simulink library "THV2THB"  (Simulink 8.2)
settings: Solver=ode45  StartTime=0.0  StopTime=10.0  RelTol=1e-3
settings Model: Creator=lena.frank  LastModifiedBy=drhf

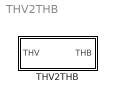
== system THV2THB ==
  THV2THB : Subsystem  InitFcn=load('THB.mat');  mask(THV2THB){}
      mask help: This block converts the old Thermo-Hydraulic-Vector to the Thermo-Hydraulic-Bus.
      mask Help: web(fullfile(path_carnot('help'),'THV2THB.html'),'-helpbrowser')

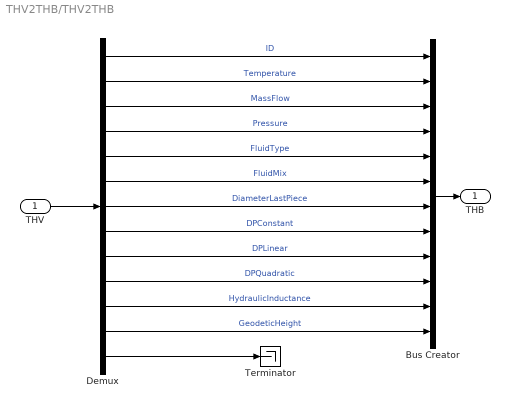
== system THV2THB/THV2THB ==
  THV : Inport
  Bus Creator : BusCreator  Inputs=12  OutDataTypeStr=Bus: THB
  Demux : Demux  Outputs=[1 1 1 1 1 1 1 1 1 1 1 1 8]
  Terminator : Terminator
  THB : Outport
  wires:
  Demux/11 -> Bus Creator/11  "HydraulicInductance"
  THV/1 -> Demux/1
  Demux/2 -> Bus Creator/2  "Temperature"
  Demux/1 -> Bus Creator/1  "ID"
  Demux/3 -> Bus Creator/3  "MassFlow"
  Demux/4 -> Bus Creator/4  "Pressure"
  Bus Creator/1 -> THB/1
  Demux/5 -> Bus Creator/5  "FluidType"
  Demux/6 -> Bus Creator/6  "FluidMix"
  Demux/7 -> Bus Creator/7  "DiameterLastPiece"
  Demux/8 -> Bus Creator/8  "DPConstant"
  Demux/9 -> Bus Creator/9  "DPLinear"
  Demux/10 -> Bus Creator/10  "DPQuadratic"
  Demux/12 -> Bus Creator/12  "GeodeticHeight"
  Demux/13 -> Terminator/1
